simulink model "slexCFunctionAdder"  (R2021a)
settings: Solver=FixedStepDiscrete  StartTime=0.0  StopTime=10  FixedStep=0.1  RelTol=1e-3  EnableMultiTasking=on
undefined symbols (not defined in the file or in its folder): deleteAdder, myAdder
Description:
  | C++ Object Methods
settings Model: ExtModeAutoUpdateStatusClock=off  Creator=The MathWorks, Inc.  LastModifiedBy=kitaw
settings SolverCC: AlgebraicLoopSolver=TrustRegion
settings DataIOCC: LimitDataPoints=on  SaveFormat=Array  SaveOutput=off  SaveTime=off  SignalLoggingName=logsOut
settings OptimizationCC: DefaultParameterBehavior=Inlined  InlineInvariantSignals=on  ExpressionDepthLimit=2147483647  EfficientFloat2IntCast=on
settings DebuggingCC: SaveWithParameterizedLinksMsg=none  SignalResolutionControl=TryResolveAllWithWarning  MultiTaskDSMMsg=warning  MultiTaskCondExecSysMsg=none  FcnCallInpInsideContextMsg=warning  StateNameClashWarn=warning  SFUnexpectedBacktrackingDiag=warning  SFNoUnconditionalDefaultTransitionDiag=warning  SFExecutionAtInitializationDiag=none  SFMachineParentedDataDiag=warning  ArithmeticOperatorsInVariantConditions=warning
settings HardwareCC: ProdBitPerPointer=32  ProdBitPerSizeT=32  ProdBitPerPtrDiffT=32  ProdLargestAtomicFloat=None  ProdIntDivRoundTo=Undefined  ProdEndianess=Unspecified  ProdWordSize=32  ProdHWDeviceType=32-bit Generic  TargetBitPerPointer=64  TargetBitPerSizeT=64  TargetBitPerPtrDiffT=64  TargetLongLongMode=on  TargetIntDivRoundTo=Zero  TargetEndianess=LittleEndian  TargetWordSize=64  TargetHWDeviceType=MATLAB Host  ProdEqTarget=off
settings ModelReferenceCC: ModelReferenceNumInstancesAllowed=Zero  PropagateSignalLabelsOutOfModel=off
settings SFSimCC: SimCustomHeaderCode="#include \"adder_cpp.h\""  SimUserSources=adder_cpp.cpp  SimUseLocalCustomCode=off  MATLABDynamicMemAlloc=off  CustomCodeUndefinedFunction=UseInterfaceOnly  SimTargetLang=C++
settings RTWCC: Description=Generic Real-Time Target  TLCOptions=-aIncludeERTFirstTime=0  GenerateReport=on  RTWUseLocalCustomCode=off  RTWUseSimCustomCode=on  CustomHeaderCode="#include \"adder_cpp.h\""  CustomSource=adder_cpp.cpp  LaunchReport=on  TargetLang=C++
settings CodeAppCC: StateflowObjectComments=on
settings GRTTargetCC: TargetLangStandard=C89/C90 (ANSI)  MatFileLogging=off
settings ConfigComp: CovMetricSettings=dw  CovSaveCumulativeToWorkspaceVar=on  CovSaveSingleToWorkspaceVar=on  CovExternalEMLEnable=off

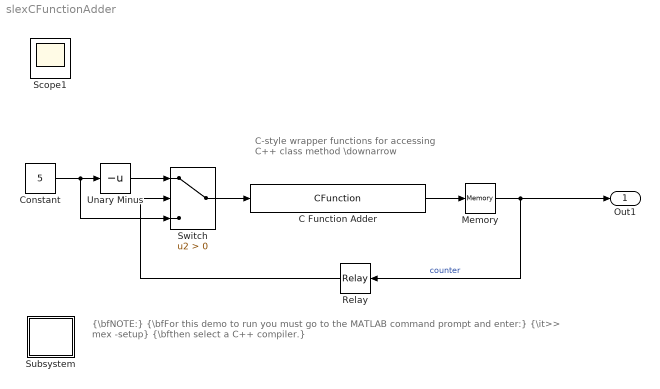
== system slexCFunctionAdder ==
  note: C-style wrapper functions for
      | accessing C++ class method
      | \downarrow
  note: {\bfNOTE:}
      | {\bfFor this demo to run you must go to the MATLAB command prompt and enter:} {\it>> mex -setup}
      | {\bfthen select a C++ compiler.}
  C Function Adder : CFunction  OutputCode=output = adderOutput(myAdder, increment);  TerminateCode=deleteAdder(myAdder);  StartCode=myAdder = createAdder();
  Constant : Constant  Value=5  OutDataTypeStr=int32
  Memory : Memory  InheritSampleTime=on  StateName=memCounter
  Relay : Relay  OnSwitchValue=101  OffSwitchValue=-1
  Subsystem : Subsystem
      mask init:
      | pos    = get_param(gcb, 'Position');
      | width  = pos(3) - pos(1);
      | height = pos(4) - pos(2);
      | 
      | marginPercent = 20;
      | marginPixels  = round(marginPercent / 100 * width);
      | 
      | x1 = width - marginPixels;
      | y1 = height;
      | x2 = width;
      | y2 = height - marginPixels;
      | x3 = width;
      | y3 = marginPixels;
      | x4 = width - marginPixels;
      | y4 = 0;
      | x5 = marginPixels;
      | y5 = 0;
      | x6 = 0;
      | y6 = marginPixels;
      | x7 = 0;
      | y7 = height - marginPixels;
      | x8 = marginPixels;
      | y8 = height;
      | 
      | xvec = [x1, x2, x3, x4, x5, x6, x7, x8];
      | yvec = [y1, y2, y3, y4, y5, y6, y7, y8];
      mask Display:
      | color('red');
      | patch(xvec, yvec);
      | color('white');
      | disp('!');
  Switch : Switch  Criteria=u2 > Threshold  ZeroCross=off
  Unary Minus : UnaryMinus
  Out1 : Outport  VectorParamsAs1DForOutWhenUnconnected=off
  Scope1 : Scope
  wires:
  Constant/1 -> Unary Minus/1, Switch/3
  Switch/1 -> C Function Adder/1
  C Function Adder/1 -> Memory/1
  Unary Minus/1 -> Switch/1
  Relay/1 -> Switch/2
  Memory/1 -> Out1/1, Relay/1  "counter"

== system slexCFunctionAdder/Subsystem ==
